simulink model "MotorDrivetuning"  (Simulink 7.4)
settings: Solver=ode45  StartTime=0.0  StopTime=60  RelTol=1e-3
undefined symbols (not defined in the file or in its folder): magnitude
libraries: simulink x1
settings Model: Creator=Rabbitfox  LastModifiedBy=Rabbitfox
settings SolverCC: ZeroCrossAlgorithm=Adaptive

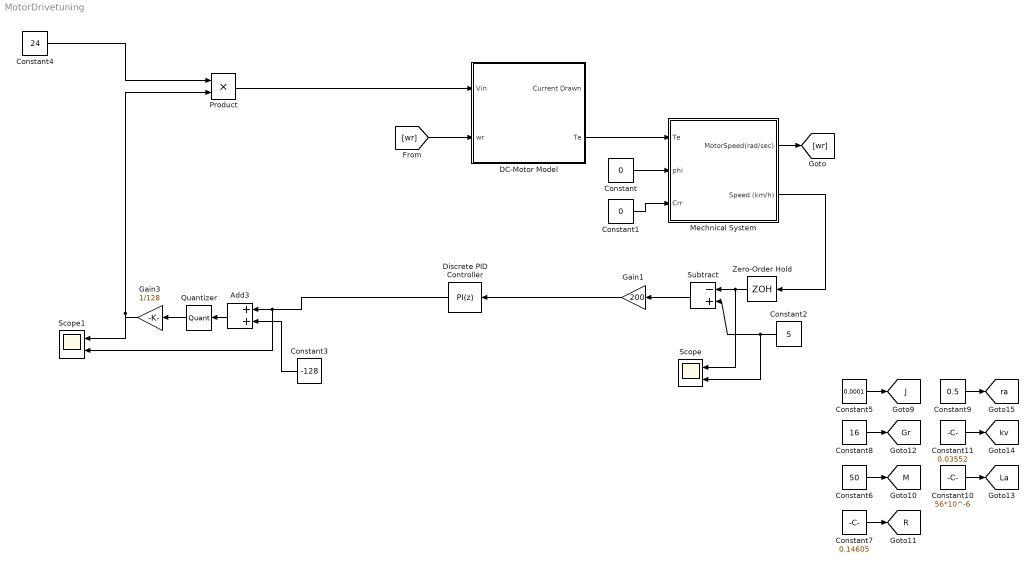
== system MotorDrivetuning ==
  Add3 : Sum  OutDataType=fixdt(1, 16)  OutScaling=2^-10
  Constant : Constant  Value=0  OutDataType=fixdt(1, 16)  OutScaling=2^0
  Constant1 : Constant  Value=0  OutDataType=fixdt(1, 16)  OutScaling=2^0
  Constant10 : Constant  Value=56*10^-6  OutDataType=fixdt(1, 16)  OutScaling=2^0
  Constant11 : Constant  Value=0.03552  OutDataType=fixdt(1, 16)  OutScaling=2^0
  Constant2 : Constant  Value=5  OutDataType=fixdt(1, 16)  OutScaling=2^0
  Constant3 : Constant  Value=-128  OutDataType=fixdt(1, 16)  OutScaling=2^0
  Constant4 : Constant  Value=24  OutDataType=fixdt(1, 16)  OutScaling=2^0
  Constant5 : Constant  Value=0.0001  OutDataType=fixdt(1, 16)  OutScaling=2^0
  Constant6 : Constant  Value=50  OutDataType=fixdt(1, 16)  OutScaling=2^0
  Constant7 : Constant  Value=0.14605  OutDataType=fixdt(1, 16)  OutScaling=2^0
  Constant8 : Constant  Value=16  OutDataType=fixdt(1, 16)  OutScaling=2^0
  Constant9 : Constant  Value=0.5  OutDataType=fixdt(1, 16)  OutScaling=2^0
  DC-Motor Model : Subsystem
  Discrete PID Controller : simulink/Continuous/PID Controller  DialogController=pidpack.PIDConfig.pidDDGCreate  DialogControllerArgs=DataTag0  SystemSampleTime=-1  Controller=PI  TimeDomain=Discrete-time  SampleTime=0.03  IntegratorMethod=Backward Euler  FilterMethod=Forward Euler  Form=Parallel  P=6.77465879799663  I=13.7879919823078  D=0  N=100  InitialConditionSource=internal  InitialConditionForIntegrator=0  InitialConditionForFilter=0  ExternalReset=none  LimitOutput=off  UpperSaturationLimit=inf  LowerSaturationLimit=-inf  LinearizeAsGain=off  AntiWindupMode=none  Kb=1  TrackingMode=off  Kt=1  PParamMin=[]  PParamMax=[]  IParamMin=[]  IParamMax=[]  DParamMin=[]  DParamMax=[]  NParamMin=[]  NParamMax=[]  KbParamMin=[]  KbParamMax=[]  KtParamMin=[]  KtParamMax=[]  POutMin=[]  POutMax=[]  IOutMin=[]  IOutMax=[]  DOutMin=[]  DOutMax=[]  NOutMin=[]  NOutMax=[]  KbOutMin=[]  KbOutMax=[]  KtOutMin=[]  KtOutMax=[]  IntegratorOutMin=[]  IntegratorOutMax=[]  FilterOutMin=[]  FilterOutMax=[]  SumOutMin=[]  SumOutMax=[]  SumI1OutMin=[]  SumI1OutMax=[]  SumI2OutMin=[]  SumI2OutMax=[]  SumI3OutMin=[]  SumI3OutMax=[]  SumDOutMin=[]  SumDOutMax=[]  SaturationOutMin=[]  SaturationOutMax=[]  IntegratorContinuousStateAttributes=''  IntegratorStateMustResolveToSignalObject=off  IntegratorRTWStateStorageClass=Auto  FilterContinuousStateAttributes=''  FilterStateMustResolveToSignalObject=off  FilterRTWStateStorageClass=Auto
  Gain1 : Gain  Gain=200  ParameterDataType=fixdt(1, 16)  ParameterScaling=2^0  OutDataType=fixdt(1, 16)  OutScaling=2^0
  Gain3 : Gain  Gain=1/128  ParameterDataType=fixdt(1, 16)  ParameterScaling=2^0  OutDataType=fixdt(1, 16)  OutScaling=2^0
  Mechnical System : Subsystem
  Product : Product  OutDataType=fixdt(1, 16)  OutScaling=2^0  RndMeth=Zero
  Quantizer : Quantizer  QuantizationInterval=1
  Scope : Scope  NumInputPorts=2
      settings: YMin=-0.001~5  YMax=0.007~5
  Scope1 : Scope  NumInputPorts=2
      settings: YMin=0.21875~155.656  YMax=0.21875~155.656
  Subtract : Sum  Inputs=-+  OutDataType=fixdt(1, 16)  OutScaling=2^-10
  Zero-Order Hold : ZeroOrderHold  SampleTime=0.03
  tag scope: Gr=global, J=global, La=global, M=global, R=global, kv=global, ra=global
  wires:
  DC-Motor Model/2(Te) -> Mechnical System/1(Te)
  Constant/1 -> Mechnical System/2(phi)
  Constant1/1 -> Mechnical System/3(Crr)
  [wr] -> DC-Motor Model/2(wr)
  Mechnical System/1(MotorSpeed(rad/sec)) -> [wr]
  Mechnical System/2(Speed (km/h)) -> Zero-Order Hold/1
  Zero-Order Hold/1 -> Subtract/1, Scope/1
  Constant2/1 -> Subtract/2, Scope/2
  Constant3/1 -> Add3/2
  Add3/1 -> Quantizer/1
  Quantizer/1 -> Gain3/1
  Product/1 -> DC-Motor Model/1(Vin)
  Gain3/1 -> Product/2, Scope1/1
  Constant4/1 -> Product/1
  Discrete PID Controller/1 -> Add3/1, Scope1/2
  Constant5/1 -> [J]
  Constant6/1 -> [M]
  Constant7/1 -> [R]
  Constant8/1 -> [Gr]
  Constant9/1 -> [ra]
  Constant10/1 -> [La]
  Constant11/1 -> [kv]
  Subtract/1 -> Gain1/1
  Gain1/1 -> Discrete PID Controller/1

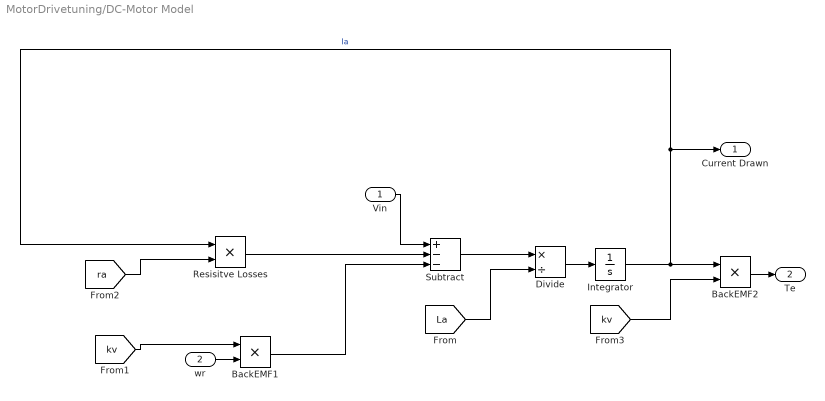
== system MotorDrivetuning/DC-Motor Model ==
  Vin : Inport
  wr : Inport  Port=2
  BackEMF1 : Product  OutDataType=fixdt(1, 16)  OutScaling=2^0  RndMeth=Zero
  BackEMF2 : Product  OutDataType=fixdt(1, 16)  OutScaling=2^0  RndMeth=Zero
  Divide : Product  Inputs=*/  OutDataType=fixdt(1, 16)  OutScaling=2^-10
  Integrator : Integrator  UpperSaturationLimit=10  LowerSaturationLimit=-10
  Resisitve Losses : Product  OutDataType=fixdt(1, 16)  OutScaling=2^0  RndMeth=Zero
  Subtract : Sum  Inputs=+--  OutDataType=fixdt(1, 16)  OutScaling=2^-10
  Current Drawn : Outport
  Te : Outport  Port=2
  wires:
  Integrator/1 -> Current Drawn/1, Resisitve Losses/1, BackEMF2/1  "Ia"
  Divide/1 -> Integrator/1
  Subtract/1 -> Divide/1
  BackEMF1/1 -> Subtract/3
  Resisitve Losses/1 -> Subtract/2
  [La] -> Divide/2
  [ra] -> Resisitve Losses/2
  [kv] -> BackEMF1/1
  Vin/1 -> Subtract/1
  wr/1 -> BackEMF1/2
  [kv] -> BackEMF2/2
  BackEMF2/1 -> Te/1

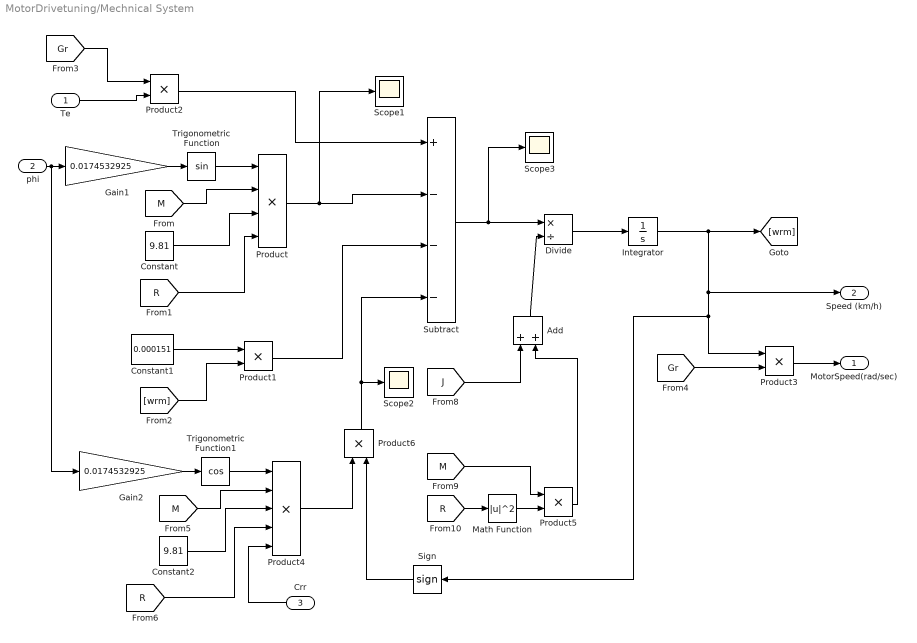
== system MotorDrivetuning/Mechnical System ==
  Te : Inport  OutDataType=fixdt(1, 16)  OutScaling=2^0
  phi : Inport  Port=2  OutDataType=fixdt(1, 16)  OutScaling=2^0
  Crr : Inport  Port=3  OutDataType=fixdt(1, 16)  OutScaling=2^0
  Add : Sum  OutDataType=fixdt(1, 16)  OutScaling=2^-10
  Constant : Constant  Value=9.81  OutDataType=fixdt(1, 16)  OutScaling=2^0
  Constant1 : Constant  Value=0.000151  OutDataType=fixdt(1, 16)  OutScaling=2^0
  Constant2 : Constant  Value=9.81  OutDataType=fixdt(1, 16)  OutScaling=2^0
  Divide : Product  Inputs=*/  OutDataType=fixdt(1, 16)  OutScaling=2^-10
  Gain1 : Gain  Gain=0.0174532925  ParameterDataType=fixdt(1, 16)  ParameterScaling=2^0  OutDataType=fixdt(1, 16)  OutScaling=2^0
  Gain2 : Gain  Gain=0.0174532925  ParameterDataType=fixdt(1, 16)  ParameterScaling=2^0  OutDataType=fixdt(1, 16)  OutScaling=2^0
  Integrator : Integrator  InitialCondition=2
  Math Function : Math  Operator=magnitude^2  OutDataType=fixdt(1, 16)  OutScaling=2^0  SaturateOnIntegerOverflow=on
  Product : Product  Inputs=4  OutDataType=fixdt(1, 16)  OutScaling=2^0  RndMeth=Zero
  Product{1..3,5..6} (5 alike) : Product  OutDataType=fixdt(1, 16)  OutScaling=2^0  RndMeth=Zero
  Product4 : Product  Inputs=5  OutDataType=fixdt(1, 16)  OutScaling=2^0  RndMeth=Zero
  Scope1 : Scope
      settings: TimeRange=10  YMin=-1  YMax=1  SaveName=ScopeData5
  Scope2 : Scope
      settings: YMin=1.776  YMax=1.7767  SaveName=ScopeData6
  Scope3 : Scope
      settings: YMin=1.776  YMax=1.7767  SaveName=ScopeData4
  Sign : Signum
  Subtract : Sum  Inputs=+---  OutDataType=fixdt(1, 16)  OutScaling=2^-10
  Trigonometric Function : Trigonometry
  Trigonometric Function1 : Trigonometry  Operator=cos
  MotorSpeed(rad/sec) : Outport  OutDataType=fixdt(1, 16)  OutScaling=2^0
  Speed (km/h) : Outport  Port=2  OutDataType=fixdt(1, 16)  OutScaling=2^0
  wires:
  Te/1 -> Product2/2
  phi/1 -> Gain1/1, Gain2/1
  Gain1/1 -> Trigonometric Function/1
  Trigonometric Function/1 -> Product/1
  [M] -> Product/2
  Constant/1 -> Product/3
  [R] -> Product/4
  Constant1/1 -> Product1/1
  Integrator/1 -> [wrm], Product3/1, Sign/1, Speed (km/h)/1
  [wrm] -> Product1/2
  [Gr] -> Product2/1
  [Gr] -> Product3/2
  Product3/1 -> MotorSpeed(rad/sec)/1
  Gain2/1 -> Trigonometric Function1/1
  Trigonometric Function1/1 -> Product4/1
  [M] -> Product4/2
  Constant2/1 -> Product4/3
  [R] -> Product4/4
  Crr/1 -> Product4/5
  Product2/1 -> Subtract/1
  Product/1 -> Subtract/2, Scope1/1
  Product1/1 -> Subtract/3
  Subtract/1 -> Divide/1, Scope3/1
  Divide/1 -> Integrator/1
  [R] -> Math Function/1
  Math Function/1 -> Product5/2
  [M] -> Product5/1
  [J] -> Add/1
  Product5/1 -> Add/2
  Add/1 -> Divide/2
  Product4/1 -> Product6/1
  Sign/1 -> Product6/2
  Product6/1 -> Subtract/4, Scope2/1
